simulink model "umich_2d_walking"  (R2012b)
settings: Solver=ode3  StartTime=0.0  StopTime=inf  FixedStep=sample_time  RelTol=1e-3
values from neighbouring files (symbols this model uses):
  fcut_unwrap = 50    [init_umich_2d_walking.m]
  fcut_velocity = 100    [init_umich_2d_walking.m]
  sample_time = 1/update_freq    (= 0.001)    [init_umich_2d_walking.m]
undefined symbols (not defined in the file or in its folder): BOOM_MAX_ENCODER_TICKS, boom_mount_angle, BOOM_PITCH_CAL_VALUE_RAD, BOOM_PITCH_CAL_VALUE_TICKS, BOOM_PITCH_ENCODER_RAD_PER_TICK, BOOM_ROLL_CAL_VALUE_RAD, BOOM_ROLL_CAL_VALUE_TICKS, BOOM_ROLL_ENCODER_RAD_PER_TICK, BOOM_YAW_ENCODER_RAD_PER_TICK, control_start_time, desired_torso_pitch, DiscIntNeverNeededParam, fcut_acceleration, gd, get, h_alpha, HIP_ABS_ENCODER_RAD_PER_TICK, hip_gravity_compensation, HIP_INC_ENCODER_RAD_PER_TICK, HIP_INC_MAX_ENCODER_TICKS, HIP_MOTOR_CONSTANT, HIP_MTR_GEAR_RATIO, HIP_MTR_MAX_TORQUE, i_limit_lateral, j_motor_reflected, k_leg_spring, kd_lateral, kd_pitch, kd_sea_torque, ki_lateral, kp_lateral, kp_pitch, kp_sea_torque, lateral_torque_ramp_time, LEFT_HIP_CALIB_POS, LEFT_HIP_CALIB_VAL, LEFT_MOTOR_HIP_DIRECTION, LEG1_LEG_A_CALIB_VAL, LEG1_LEG_A_RAD_PER_CNT, LEG1_LEG_B_CALIB_VAL, LEG1_LEG_B_RAD_PER_CNT, LEG1_MOTOR_A_DIRECTION, LEG1_MOTOR_B_DIRECTION, LEG1_TRAN_A_CALIB_VAL, LEG1_TRAN_A_RAD_PER_CNT, LEG1_TRAN_B_CALIB_VAL, LEG1_TRAN_B_RAD_PER_CNT, LEG2_LEG_A_CALIB_VAL, LEG2_LEG_A_RAD_PER_CNT, LEG2_LEG_B_CALIB_VAL, LEG2_LEG_B_RAD_PER_CNT, LEG2_MOTOR_A_DIRECTION, LEG2_MOTOR_B_DIRECTION, LEG2_TRAN_A_CALIB_VAL, LEG2_TRAN_A_RAD_PER_CNT, LEG2_TRAN_B_CALIB_VAL, LEG2_TRAN_B_RAD_PER_CNT, LEG_A_CALIB_LOC, LEG_B_CALIB_LOC, LEG_MOTOR_CONSTANT ... (+23)
libraries: xpcethercatlib x160, simulink x9, dspswit3 x1
(part 2 of 3)

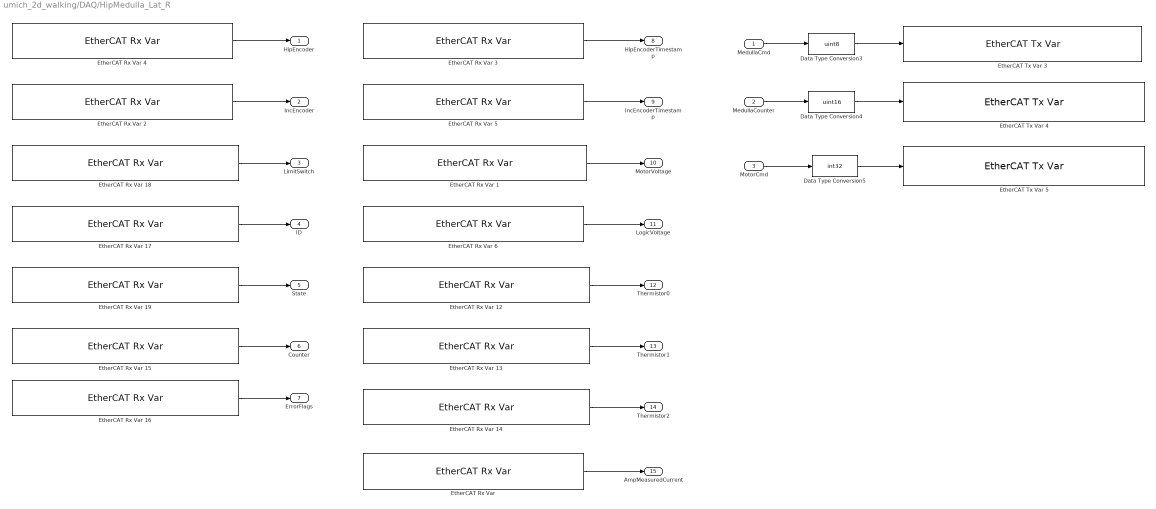
== system umich_2d_walking/DAQ/HipMedulla_Lat_R ==
  MedullaCmd : Inport
  MedullaCounter : Inport  Port=2
  MotorCmd : Inport  Port=3
  Data Type Conversion3 : DataTypeConversion  OutDataTypeStr=uint8
  Data Type Conversion4 : DataTypeConversion  OutDataTypeStr=uint16
  Data Type Conversion5 : DataTypeConversion  OutDataTypeStr=int32
  "EtherCAT Rx Var " : xpcethercatlib/EtherCAT Rx Var   Priority=2  sig_name=Box 6 (ATRIAS 2.1 Hip (Medulla 1.5)).Measured Current.Amp Measured Current  sig_offset=2352  sig_type=int16  type_size=16  sig_dim=1  device_id=0  sample_time=0.001000
  EtherCAT Rx Var 1 : xpcethercatlib/EtherCAT Rx Var   Priority=2  sig_name=Box 6 (ATRIAS 2.1 Hip (Medulla 1.5)).Power.Motor Voltage  sig_offset=2272  sig_type=uint16  type_size=16  sig_dim=1  device_id=0  sample_time=0.001000
  EtherCAT Rx Var 12 : xpcethercatlib/EtherCAT Rx Var   Priority=2  sig_name=Box 6 (ATRIAS 2.1 Hip (Medulla 1.5)).Thermistors.Thermistor 0  sig_offset=2304  sig_type=uint16  type_size=16  sig_dim=1  device_id=0  sample_time=0.001000
  EtherCAT Rx Var 13 : xpcethercatlib/EtherCAT Rx Var   Priority=2  sig_name=Box 6 (ATRIAS 2.1 Hip (Medulla 1.5)).Thermistors.Thermistor 1  sig_offset=2320  sig_type=uint16  type_size=16  sig_dim=1  device_id=0  sample_time=0.001000
  EtherCAT Rx Var 14 : xpcethercatlib/EtherCAT Rx Var   Priority=2  sig_name=Box 6 (ATRIAS 2.1 Hip (Medulla 1.5)).Thermistors.Thermistor 2  sig_offset=2336  sig_type=uint16  type_size=16  sig_dim=1  device_id=0  sample_time=0.001000
  EtherCAT Rx Var 15 : xpcethercatlib/EtherCAT Rx Var   Priority=2  sig_name=Box 6 (ATRIAS 2.1 Hip (Medulla 1.5)).uController Status.Counter  sig_offset=2200  sig_type=uint8  type_size=8  sig_dim=1  device_id=0  sample_time=0.001000
  EtherCAT Rx Var 16 : xpcethercatlib/EtherCAT Rx Var   Priority=2  sig_name=Box 6 (ATRIAS 2.1 Hip (Medulla 1.5)).uController Status.Error Flags  sig_offset=2208  sig_type=uint8  type_size=8  sig_dim=1  device_id=0  sample_time=0.001000
  EtherCAT Rx Var 17 : xpcethercatlib/EtherCAT Rx Var   Priority=2  sig_name=Box 6 (ATRIAS 2.1 Hip (Medulla 1.5)).uController Status.ID  sig_offset=2184  sig_type=uint8  type_size=8  sig_dim=1  device_id=0  sample_time=0.001000
  EtherCAT Rx Var 18 : xpcethercatlib/EtherCAT Rx Var   Priority=2  sig_name=Box 6 (ATRIAS 2.1 Hip (Medulla 1.5)).uController Status.Limit Switch  sig_offset=2216  sig_type=uint8  type_size=8  sig_dim=1  device_id=0  sample_time=0.001000
  EtherCAT Rx Var 19 : xpcethercatlib/EtherCAT Rx Var   Priority=2  sig_name=Box 6 (ATRIAS 2.1 Hip (Medulla 1.5)).uController Status.State  sig_offset=2192  sig_type=uint8  type_size=8  sig_dim=1  device_id=0  sample_time=0.001000
  EtherCAT Rx Var 2 : xpcethercatlib/EtherCAT Rx Var   Priority=2  sig_name=Box 6 (ATRIAS 2.1 Hip (Medulla 1.5)).Incremental Encoder.Incremental Encoder  sig_offset=2368  sig_type=uint16  type_size=16  sig_dim=1  device_id=0  sample_time=0.001000
  EtherCAT Rx Var 3 : xpcethercatlib/EtherCAT Rx Var   Priority=2  sig_name=Box 6 (ATRIAS 2.1 Hip (Medulla 1.5)).Hip Encoder.Timestamp  sig_offset=2256  sig_type=uint16  type_size=16  sig_dim=1  device_id=0  sample_time=0.001000
  EtherCAT Rx Var 4 : xpcethercatlib/EtherCAT Rx Var   Priority=2  sig_name=Box 6 (ATRIAS 2.1 Hip (Medulla 1.5)).Hip Encoder.Encoder  sig_offset=2224  sig_type=uint32  type_size=32  sig_dim=1  device_id=0  sample_time=0.001000
  EtherCAT Rx Var 5 : xpcethercatlib/EtherCAT Rx Var   Priority=2  sig_name=Box 6 (ATRIAS 2.1 Hip (Medulla 1.5)).Incremental Encoder.Incremental Encoder Timestamp  sig_offset=2384  sig_type=uint16  type_size=16  sig_dim=1  device_id=0  sample_time=0.001000
  EtherCAT Rx Var 6 : xpcethercatlib/EtherCAT Rx Var   Priority=2  sig_name=Box 6 (ATRIAS 2.1 Hip (Medulla 1.5)).Power.Logic Voltage  sig_offset=2288  sig_type=uint16  type_size=16  sig_dim=1  device_id=0  sample_time=0.001000
  EtherCAT Tx Var 3 : xpcethercatlib/EtherCAT Tx Var   Priority=3  sig_name=Box 6 (ATRIAS 2.1 Hip (Medulla 1.5)).uControllerInput.Command  sig_offset=2184  sig_type=uint8  type_size=8  sig_dim=1  device_id=0  sample_time=0.001000
  EtherCAT Tx Var 4 : xpcethercatlib/EtherCAT Tx Var   Priority=3  sig_name=Box 6 (ATRIAS 2.1 Hip (Medulla 1.5)).uControllerInput.Counter  sig_offset=2192  sig_type=uint16  type_size=16  sig_dim=1  device_id=0  sample_time=0.001000
  EtherCAT Tx Var 5 : xpcethercatlib/EtherCAT Tx Var   Priority=3  sig_name=Box 6 (ATRIAS 2.1 Hip (Medulla 1.5)).uControllerInput.Motor Current  sig_offset=2208  sig_type=int32  type_size=32  sig_dim=1  device_id=0  sample_time=0.001000
  HipEncoder : Outport
  IncEncoder : Outport  Port=2
  LimitSwitch : Outport  Port=3
  ID : Outport  Port=4
  State : Outport  Port=5
  Counter : Outport  Port=6
  ErrorFlags : Outport  Port=7
  HipEncoderTimestamp : Outport  Port=8
  IncEncoderTimestamp : Outport  Port=9
  MotorVoltage : Outport  Port=10
  LogicVoltage : Outport  Port=11
  Thermistor0 : Outport  Port=12
  Thermistor1 : Outport  Port=13
  Thermistor2 : Outport  Port=14
  AmpMeasuredCurrent : Outport  Port=15
  wires:
  Data Type Conversion3/1 -> EtherCAT Tx Var 3/1
  Data Type Conversion4/1 -> EtherCAT Tx Var 4/1
  Data Type Conversion5/1 -> EtherCAT Tx Var 5/1
  MedullaCmd/1 -> Data Type Conversion3/1
  MedullaCounter/1 -> Data Type Conversion4/1
  MotorCmd/1 -> Data Type Conversion5/1
  EtherCAT Rx Var 5/1 -> IncEncoderTimestamp/1
  EtherCAT Rx Var 4/1 -> HipEncoder/1
  EtherCAT Rx Var 3/1 -> HipEncoderTimestamp/1
  EtherCAT Rx Var 2/1 -> IncEncoder/1
  EtherCAT Rx Var 15/1 -> Counter/1
  EtherCAT Rx Var 17/1 -> ID/1
  EtherCAT Rx Var 18/1 -> LimitSwitch/1
  EtherCAT Rx Var 19/1 -> State/1
  EtherCAT Rx Var 16/1 -> ErrorFlags/1
  EtherCAT Rx Var 6/1 -> LogicVoltage/1
  EtherCAT Rx Var 1/1 -> MotorVoltage/1
  EtherCAT Rx Var 12/1 -> Thermistor0/1
  EtherCAT Rx Var 13/1 -> Thermistor1/1
  EtherCAT Rx Var 14/1 -> Thermistor2/1
  "EtherCAT Rx Var "/1 -> AmpMeasuredCurrent/1

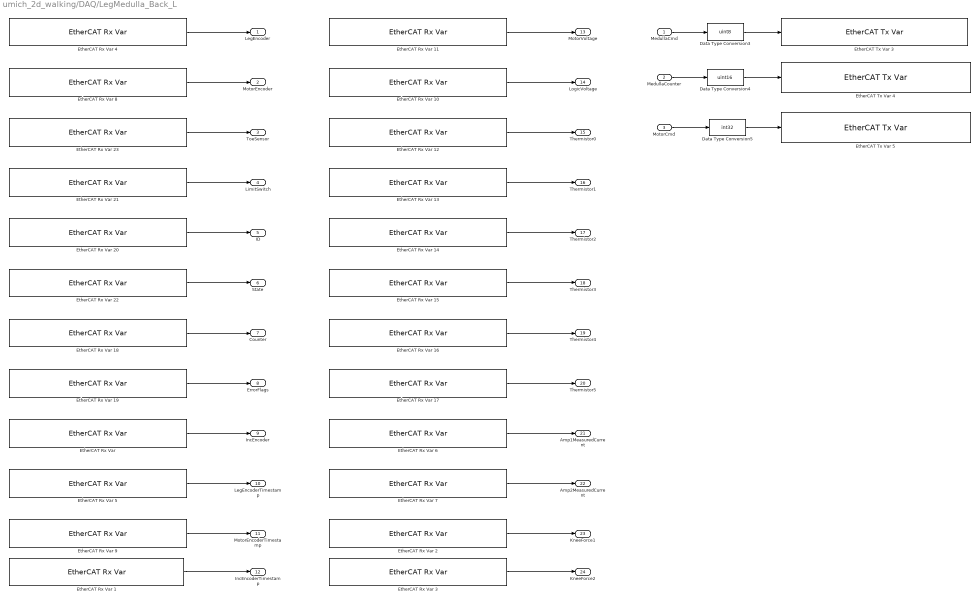
== system umich_2d_walking/DAQ/LegMedulla_Back_L ==
  MedullaCmd : Inport
  MedullaCounter : Inport  Port=2
  MotorCmd : Inport  Port=3
  Data Type Conversion3 : DataTypeConversion  OutDataTypeStr=uint8
  Data Type Conversion4 : DataTypeConversion  OutDataTypeStr=uint16
  Data Type Conversion5 : DataTypeConversion  OutDataTypeStr=int32
  "EtherCAT Rx Var " : xpcethercatlib/EtherCAT Rx Var   Priority=2  sig_name=Box 3 (ATRIAS 2.1 Leg (Medulla 1.5)).Incremental Encoder.Incremental Encoder  sig_offset=1368  sig_type=uint16  type_size=16  sig_dim=1  device_id=0  sample_time=0.001000
  EtherCAT Rx Var 1 : xpcethercatlib/EtherCAT Rx Var   Priority=2  sig_name=Box 3 (ATRIAS 2.1 Leg (Medulla 1.5)).Incremental Encoder.Incremental Encoder Timestamp  sig_offset=1384  sig_type=uint16  type_size=16  sig_dim=1  device_id=0  sample_time=0.001000
  EtherCAT Rx Var 10 : xpcethercatlib/EtherCAT Rx Var   Priority=2  sig_name=Box 3 (ATRIAS 2.1 Leg (Medulla 1.5)).Power.Logic Voltage  sig_offset=1416  sig_type=uint16  type_size=16  sig_dim=1  device_id=0  sample_time=0.001000
  EtherCAT Rx Var 11 : xpcethercatlib/EtherCAT Rx Var   Priority=2  sig_name=Box 3 (ATRIAS 2.1 Leg (Medulla 1.5)).Power.Motor Voltage  sig_offset=1400  sig_type=uint16  type_size=16  sig_dim=1  device_id=0  sample_time=0.001000
  EtherCAT Rx Var 12 : xpcethercatlib/EtherCAT Rx Var   Priority=2  sig_name=Box 3 (ATRIAS 2.1 Leg (Medulla 1.5)).Thermistors.Thermistor 0  sig_offset=1432  sig_type=uint16  type_size=16  sig_dim=1  device_id=0  sample_time=0.001000
  EtherCAT Rx Var 13 : xpcethercatlib/EtherCAT Rx Var   Priority=2  sig_name=Box 3 (ATRIAS 2.1 Leg (Medulla 1.5)).Thermistors.Thermistor 1  sig_offset=1448  sig_type=uint16  type_size=16  sig_dim=1  device_id=0  sample_time=0.001000
  EtherCAT Rx Var 14 : xpcethercatlib/EtherCAT Rx Var   Priority=2  sig_name=Box 3 (ATRIAS 2.1 Leg (Medulla 1.5)).Thermistors.Thermistor 2  sig_offset=1464  sig_type=uint16  type_size=16  sig_dim=1  device_id=0  sample_time=0.001000
  EtherCAT Rx Var 15 : xpcethercatlib/EtherCAT Rx Var   Priority=2  sig_name=Box 3 (ATRIAS 2.1 Leg (Medulla 1.5)).Thermistors.Thermistor 3  sig_offset=1480  sig_type=uint16  type_size=16  sig_dim=1  device_id=0  sample_time=0.001000
  EtherCAT Rx Var 16 : xpcethercatlib/EtherCAT Rx Var   Priority=2  sig_name=Box 3 (ATRIAS 2.1 Leg (Medulla 1.5)).Thermistors.Thermistor 4  sig_offset=1496  sig_type=uint16  type_size=16  sig_dim=1  device_id=0  sample_time=0.001000
  EtherCAT Rx Var 17 : xpcethercatlib/EtherCAT Rx Var   Priority=2  sig_name=Box 3 (ATRIAS 2.1 Leg (Medulla 1.5)).Thermistors.Thermistor 5  sig_offset=1512  sig_type=uint16  type_size=16  sig_dim=1  device_id=0  sample_time=0.001000
  EtherCAT Rx Var 18 : xpcethercatlib/EtherCAT Rx Var   Priority=2  sig_name=Box 3 (ATRIAS 2.1 Leg (Medulla 1.5)).uController Status.Counter  sig_offset=1232  sig_type=uint8  type_size=8  sig_dim=1  device_id=0  sample_time=0.001000
  EtherCAT Rx Var 19 : xpcethercatlib/EtherCAT Rx Var   Priority=2  sig_name=Box 3 (ATRIAS 2.1 Leg (Medulla 1.5)).uController Status.Error Flags  sig_offset=1240  sig_type=uint8  type_size=8  sig_dim=1  device_id=0  sample_time=0.001000
  EtherCAT Rx Var 2 : xpcethercatlib/EtherCAT Rx Var   Priority=2  sig_name=Box 3 (ATRIAS 2.1 Leg (Medulla 1.5)).Knee Force.Knee Force 1  sig_offset=1560  sig_type=uint16  type_size=16  sig_dim=1  device_id=0  sample_time=0.001000
  EtherCAT Rx Var 20 : xpcethercatlib/EtherCAT Rx Var   Priority=2  sig_name=Box 3 (ATRIAS 2.1 Leg (Medulla 1.5)).uController Status.ID  sig_offset=1216  sig_type=uint8  type_size=8  sig_dim=1  device_id=0  sample_time=0.001000
  EtherCAT Rx Var 21 : xpcethercatlib/EtherCAT Rx Var   Priority=2  sig_name=Box 3 (ATRIAS 2.1 Leg (Medulla 1.5)).uController Status.Limit Switch  sig_offset=1248  sig_type=uint8  type_size=8  sig_dim=1  device_id=0  sample_time=0.001000
  EtherCAT Rx Var 22 : xpcethercatlib/EtherCAT Rx Var   Priority=2  sig_name=Box 3 (ATRIAS 2.1 Leg (Medulla 1.5)).uController Status.State  sig_offset=1224  sig_type=uint8  type_size=8  sig_dim=1  device_id=0  sample_time=0.001000
  EtherCAT Rx Var 23 : xpcethercatlib/EtherCAT Rx Var   Priority=2  sig_name=Box 3 (ATRIAS 2.1 Leg (Medulla 1.5)).uController Status.Toe Sensor  sig_offset=1256  sig_type=uint16  type_size=16  sig_dim=1  device_id=0  sample_time=0.001000
  EtherCAT Rx Var 3 : xpcethercatlib/EtherCAT Rx Var   Priority=2  sig_name=Box 3 (ATRIAS 2.1 Leg (Medulla 1.5)).Knee Force.Knee Force 2  sig_offset=1576  sig_type=uint16  type_size=16  sig_dim=1  device_id=0  sample_time=0.001000
  EtherCAT Rx Var 4 : xpcethercatlib/EtherCAT Rx Var   Priority=2  sig_name=Box 3 (ATRIAS 2.1 Leg (Medulla 1.5)).Leg Encoder.Leg Encoder  sig_offset=1320  sig_type=uint32  type_size=32  sig_dim=1  device_id=0  sample_time=0.001000
  EtherCAT Rx Var 5 : xpcethercatlib/EtherCAT Rx Var   Priority=2  sig_name=Box 3 (ATRIAS 2.1 Leg (Medulla 1.5)).Leg Encoder.Leg Encoder Timestamp  sig_offset=1352  sig_type=uint16  type_size=16  sig_dim=1  device_id=0  sample_time=0.001000
  EtherCAT Rx Var 6 : xpcethercatlib/EtherCAT Rx Var   Priority=2  sig_name=Box 3 (ATRIAS 2.1 Leg (Medulla 1.5)).Measured Current.Amp 1 Measured Current  sig_offset=1528  sig_type=int16  type_size=16  sig_dim=1  device_id=0  sample_time=0.001000
  EtherCAT Rx Var 7 : xpcethercatlib/EtherCAT Rx Var   Priority=2  sig_name=Box 3 (ATRIAS 2.1 Leg (Medulla 1.5)).Measured Current.Amp 2 Measured Current  sig_offset=1544  sig_type=int16  type_size=16  sig_dim=1  device_id=0  sample_time=0.001000
  EtherCAT Rx Var 8 : xpcethercatlib/EtherCAT Rx Var   Priority=2  sig_name=Box 3 (ATRIAS 2.1 Leg (Medulla 1.5)).Motor Encoder.Motor Encoder  sig_offset=1272  sig_type=uint32  type_size=32  sig_dim=1  device_id=0  sample_time=0.001000
  EtherCAT Rx Var 9 : xpcethercatlib/EtherCAT Rx Var   Priority=2  sig_name=Box 3 (ATRIAS 2.1 Leg (Medulla 1.5)).Motor Encoder.Motor Encoder Timestamp  sig_offset=1304  sig_type=uint16  type_size=16  sig_dim=1  device_id=0  sample_time=0.001000
  EtherCAT Tx Var 3 : xpcethercatlib/EtherCAT Tx Var   Priority=3  sig_name=Box 3 (ATRIAS 2.1 Leg (Medulla 1.5)).uControllerInput.Command  sig_offset=1216  sig_type=uint8  type_size=8  sig_dim=1  device_id=0  sample_time=0.001000
  EtherCAT Tx Var 4 : xpcethercatlib/EtherCAT Tx Var   Priority=3  sig_name=Box 3 (ATRIAS 2.1 Leg (Medulla 1.5)).uControllerInput.Counter  sig_offset=1224  sig_type=uint16  type_size=16  sig_dim=1  device_id=0  sample_time=0.001000
  EtherCAT Tx Var 5 : xpcethercatlib/EtherCAT Tx Var   Priority=3  sig_name=Box 3 (ATRIAS 2.1 Leg (Medulla 1.5)).uControllerInput.Motor Current  sig_offset=1240  sig_type=int32  type_size=32  sig_dim=1  device_id=0  sample_time=0.001000
  LegEncoder : Outport
  MotorEncoder : Outport  Port=2
  ToeSensor : Outport  Port=3
  LimitSwitch : Outport  Port=4
  ID : Outport  Port=5
  State : Outport  Port=6
  Counter : Outport  Port=7
  ErrorFlags : Outport  Port=8
  IncEncoder : Outport  Port=9
  LegEncoderTimestamp : Outport  Port=10
  MotorEncoderTimestamp : Outport  Port=11
  IncEncoderTimestamp : Outport  Port=12
  MotorVoltage : Outport  Port=13
  LogicVoltage : Outport  Port=14
  Thermistor0 : Outport  Port=15
  Thermistor1 : Outport  Port=16
  Thermistor2 : Outport  Port=17
  Thermistor3 : Outport  Port=18
  Thermistor4 : Outport  Port=19
  Thermistor5 : Outport  Port=20
  Amp1MeasuredCurrent : Outport  Port=21
  Amp2MeasuredCurrent : Outport  Port=22
  KneeForce1 : Outport  Port=23
  KneeForce2 : Outport  Port=24
  wires:
  Data Type Conversion3/1 -> EtherCAT Tx Var 3/1
  Data Type Conversion4/1 -> EtherCAT Tx Var 4/1
  Data Type Conversion5/1 -> EtherCAT Tx Var 5/1
  "EtherCAT Rx Var "/1 -> IncEncoder/1
  EtherCAT Rx Var 1/1 -> IncEncoderTimestamp/1
  EtherCAT Rx Var 2/1 -> KneeForce1/1
  EtherCAT Rx Var 3/1 -> KneeForce2/1
  EtherCAT Rx Var 4/1 -> LegEncoder/1
  EtherCAT Rx Var 5/1 -> LegEncoderTimestamp/1
  EtherCAT Rx Var 6/1 -> Amp1MeasuredCurrent/1
  EtherCAT Rx Var 7/1 -> Amp2MeasuredCurrent/1
  EtherCAT Rx Var 8/1 -> MotorEncoder/1
  EtherCAT Rx Var 9/1 -> MotorEncoderTimestamp/1
  EtherCAT Rx Var 10/1 -> LogicVoltage/1
  EtherCAT Rx Var 11/1 -> MotorVoltage/1
  EtherCAT Rx Var 12/1 -> Thermistor0/1
  EtherCAT Rx Var 13/1 -> Thermistor1/1
  EtherCAT Rx Var 14/1 -> Thermistor2/1
  EtherCAT Rx Var 15/1 -> Thermistor3/1
  EtherCAT Rx Var 16/1 -> Thermistor4/1
  EtherCAT Rx Var 17/1 -> Thermistor5/1
  EtherCAT Rx Var 18/1 -> Counter/1
  EtherCAT Rx Var 19/1 -> ErrorFlags/1
  EtherCAT Rx Var 20/1 -> ID/1
  EtherCAT Rx Var 21/1 -> LimitSwitch/1
  EtherCAT Rx Var 22/1 -> State/1
  EtherCAT Rx Var 23/1 -> ToeSensor/1
  MedullaCmd/1 -> Data Type Conversion3/1
  MedullaCounter/1 -> Data Type Conversion4/1
  MotorCmd/1 -> Data Type Conversion5/1

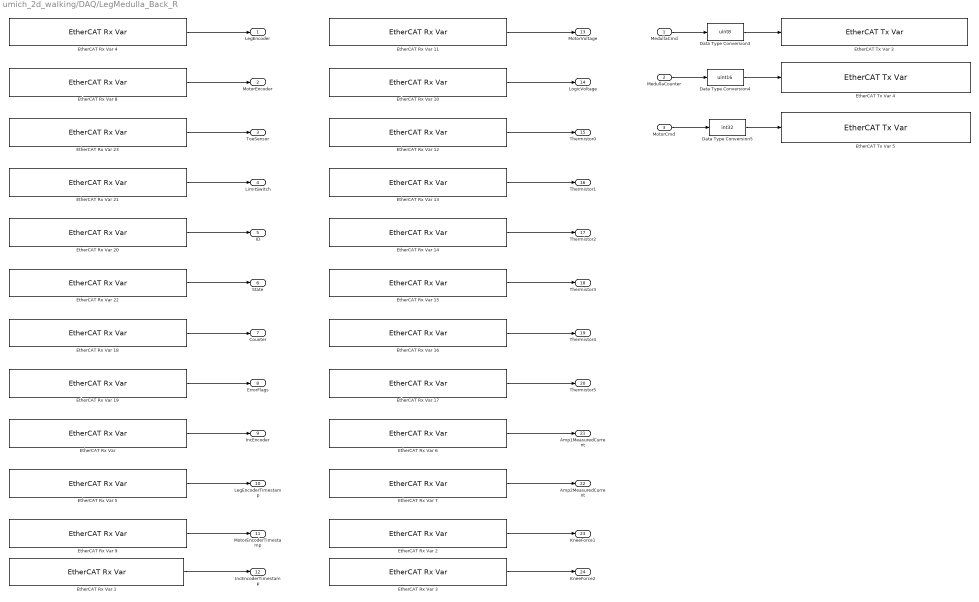
== system umich_2d_walking/DAQ/LegMedulla_Back_R ==
  MedullaCmd : Inport
  MedullaCounter : Inport  Port=2
  MotorCmd : Inport  Port=3
  Data Type Conversion3 : DataTypeConversion  OutDataTypeStr=uint8
  Data Type Conversion4 : DataTypeConversion  OutDataTypeStr=uint16
  Data Type Conversion5 : DataTypeConversion  OutDataTypeStr=int32
  "EtherCAT Rx Var " : xpcethercatlib/EtherCAT Rx Var   Priority=2  sig_name=Box 1 (ATRIAS 2.1 Leg (Medulla 1.5)).Incremental Encoder.Incremental Encoder  sig_offset=616  sig_type=uint16  type_size=16  sig_dim=1  device_id=0  sample_time=0.001000
  EtherCAT Rx Var 1 : xpcethercatlib/EtherCAT Rx Var   Priority=2  sig_name=Box 1 (ATRIAS 2.1 Leg (Medulla 1.5)).Incremental Encoder.Incremental Encoder Timestamp  sig_offset=632  sig_type=uint16  type_size=16  sig_dim=1  device_id=0  sample_time=0.001000
  EtherCAT Rx Var 10 : xpcethercatlib/EtherCAT Rx Var   Priority=2  sig_name=Box 1 (ATRIAS 2.1 Leg (Medulla 1.5)).Power.Logic Voltage  sig_offset=664  sig_type=uint16  type_size=16  sig_dim=1  device_id=0  sample_time=0.001000
  EtherCAT Rx Var 11 : xpcethercatlib/EtherCAT Rx Var   Priority=2  sig_name=Box 1 (ATRIAS 2.1 Leg (Medulla 1.5)).Power.Motor Voltage  sig_offset=648  sig_type=uint16  type_size=16  sig_dim=1  device_id=0  sample_time=0.001000
  EtherCAT Rx Var 12 : xpcethercatlib/EtherCAT Rx Var   Priority=2  sig_name=Box 1 (ATRIAS 2.1 Leg (Medulla 1.5)).Thermistors.Thermistor 0  sig_offset=680  sig_type=uint16  type_size=16  sig_dim=1  device_id=0  sample_time=0.001000
  EtherCAT Rx Var 13 : xpcethercatlib/EtherCAT Rx Var   Priority=2  sig_name=Box 1 (ATRIAS 2.1 Leg (Medulla 1.5)).Thermistors.Thermistor 1  sig_offset=696  sig_type=uint16  type_size=16  sig_dim=1  device_id=0  sample_time=0.001000
  EtherCAT Rx Var 14 : xpcethercatlib/EtherCAT Rx Var   Priority=2  sig_name=Box 1 (ATRIAS 2.1 Leg (Medulla 1.5)).Thermistors.Thermistor 2  sig_offset=712  sig_type=uint16  type_size=16  sig_dim=1  device_id=0  sample_time=0.001000
  EtherCAT Rx Var 15 : xpcethercatlib/EtherCAT Rx Var   Priority=2  sig_name=Box 1 (ATRIAS 2.1 Leg (Medulla 1.5)).Thermistors.Thermistor 3  sig_offset=728  sig_type=uint16  type_size=16  sig_dim=1  device_id=0  sample_time=0.001000
  EtherCAT Rx Var 16 : xpcethercatlib/EtherCAT Rx Var   Priority=2  sig_name=Box 1 (ATRIAS 2.1 Leg (Medulla 1.5)).Thermistors.Thermistor 4  sig_offset=744  sig_type=uint16  type_size=16  sig_dim=1  device_id=0  sample_time=0.001000
  EtherCAT Rx Var 17 : xpcethercatlib/EtherCAT Rx Var   Priority=2  sig_name=Box 1 (ATRIAS 2.1 Leg (Medulla 1.5)).Thermistors.Thermistor 5  sig_offset=760  sig_type=uint16  type_size=16  sig_dim=1  device_id=0  sample_time=0.001000
  EtherCAT Rx Var 18 : xpcethercatlib/EtherCAT Rx Var   Priority=2  sig_name=Box 1 (ATRIAS 2.1 Leg (Medulla 1.5)).uController Status.Counter  sig_offset=480  sig_type=uint8  type_size=8  sig_dim=1  device_id=0  sample_time=0.001000
  EtherCAT Rx Var 19 : xpcethercatlib/EtherCAT Rx Var   Priority=2  sig_name=Box 1 (ATRIAS 2.1 Leg (Medulla 1.5)).uController Status.Error Flags  sig_offset=488  sig_type=uint8  type_size=8  sig_dim=1  device_id=0  sample_time=0.001000
  EtherCAT Rx Var 2 : xpcethercatlib/EtherCAT Rx Var   Priority=2  sig_name=Box 1 (ATRIAS 2.1 Leg (Medulla 1.5)).Knee Force.Knee Force 1  sig_offset=808  sig_type=uint16  type_size=16  sig_dim=1  device_id=0  sample_time=0.001000
  EtherCAT Rx Var 20 : xpcethercatlib/EtherCAT Rx Var   Priority=2  sig_name=Box 1 (ATRIAS 2.1 Leg (Medulla 1.5)).uController Status.ID  sig_offset=464  sig_type=uint8  type_size=8  sig_dim=1  device_id=0  sample_time=0.001000
  EtherCAT Rx Var 21 : xpcethercatlib/EtherCAT Rx Var   Priority=2  sig_name=Box 1 (ATRIAS 2.1 Leg (Medulla 1.5)).uController Status.Limit Switch  sig_offset=496  sig_type=uint8  type_size=8  sig_dim=1  device_id=0  sample_time=0.001000
  EtherCAT Rx Var 22 : xpcethercatlib/EtherCAT Rx Var   Priority=2  sig_name=Box 1 (ATRIAS 2.1 Leg (Medulla 1.5)).uController Status.State  sig_offset=472  sig_type=uint8  type_size=8  sig_dim=1  device_id=0  sample_time=0.001000
  EtherCAT Rx Var 23 : xpcethercatlib/EtherCAT Rx Var   Priority=2  sig_name=Box 1 (ATRIAS 2.1 Leg (Medulla 1.5)).uController Status.Toe Sensor  sig_offset=504  sig_type=uint16  type_size=16  sig_dim=1  device_id=0  sample_time=0.001000
  EtherCAT Rx Var 3 : xpcethercatlib/EtherCAT Rx Var   Priority=2  sig_name=Box 1 (ATRIAS 2.1 Leg (Medulla 1.5)).Knee Force.Knee Force 2  sig_offset=824  sig_type=uint16  type_size=16  sig_dim=1  device_id=0  sample_time=0.001000
  EtherCAT Rx Var 4 : xpcethercatlib/EtherCAT Rx Var   Priority=2  sig_name=Box 1 (ATRIAS 2.1 Leg (Medulla 1.5)).Leg Encoder.Leg Encoder  sig_offset=568  sig_type=uint32  type_size=32  sig_dim=1  device_id=0  sample_time=0.001000
  EtherCAT Rx Var 5 : xpcethercatlib/EtherCAT Rx Var   Priority=2  sig_name=Box 1 (ATRIAS 2.1 Leg (Medulla 1.5)).Leg Encoder.Leg Encoder Timestamp  sig_offset=600  sig_type=uint16  type_size=16  sig_dim=1  device_id=0  sample_time=0.001000
  EtherCAT Rx Var 6 : xpcethercatlib/EtherCAT Rx Var   Priority=2  sig_name=Box 1 (ATRIAS 2.1 Leg (Medulla 1.5)).Measured Current.Amp 1 Measured Current  sig_offset=776  sig_type=int16  type_size=16  sig_dim=1  device_id=0  sample_time=0.001000
  EtherCAT Rx Var 7 : xpcethercatlib/EtherCAT Rx Var   Priority=2  sig_name=Box 1 (ATRIAS 2.1 Leg (Medulla 1.5)).Measured Current.Amp 2 Measured Current  sig_offset=792  sig_type=int16  type_size=16  sig_dim=1  device_id=0  sample_time=0.001000
  EtherCAT Rx Var 8 : xpcethercatlib/EtherCAT Rx Var   Priority=2  sig_name=Box 1 (ATRIAS 2.1 Leg (Medulla 1.5)).Motor Encoder.Motor Encoder  sig_offset=520  sig_type=uint32  type_size=32  sig_dim=1  device_id=0  sample_time=0.001000
  EtherCAT Rx Var 9 : xpcethercatlib/EtherCAT Rx Var   Priority=2  sig_name=Box 1 (ATRIAS 2.1 Leg (Medulla 1.5)).Motor Encoder.Motor Encoder Timestamp  sig_offset=552  sig_type=uint16  type_size=16  sig_dim=1  device_id=0  sample_time=0.001000
  EtherCAT Tx Var 3 : xpcethercatlib/EtherCAT Tx Var   Priority=3  sig_name=Box 1 (ATRIAS 2.1 Leg (Medulla 1.5)).uControllerInput.Command  sig_offset=464  sig_type=uint8  type_size=8  sig_dim=1  device_id=0  sample_time=0.001000
  EtherCAT Tx Var 4 : xpcethercatlib/EtherCAT Tx Var   Priority=3  sig_name=Box 1 (ATRIAS 2.1 Leg (Medulla 1.5)).uControllerInput.Counter  sig_offset=472  sig_type=uint16  type_size=16  sig_dim=1  device_id=0  sample_time=0.001000
  EtherCAT Tx Var 5 : xpcethercatlib/EtherCAT Tx Var   Priority=3  sig_name=Box 1 (ATRIAS 2.1 Leg (Medulla 1.5)).uControllerInput.Motor Current  sig_offset=488  sig_type=int32  type_size=32  sig_dim=1  device_id=0  sample_time=0.001000
  LegEncoder : Outport
  MotorEncoder : Outport  Port=2
  ToeSensor : Outport  Port=3
  LimitSwitch : Outport  Port=4
  ID : Outport  Port=5
  State : Outport  Port=6
  Counter : Outport  Port=7
  ErrorFlags : Outport  Port=8
  IncEncoder : Outport  Port=9
  LegEncoderTimestamp : Outport  Port=10
  MotorEncoderTimestamp : Outport  Port=11
  IncEncoderTimestamp : Outport  Port=12
  MotorVoltage : Outport  Port=13
  LogicVoltage : Outport  Port=14
  Thermistor0 : Outport  Port=15
  Thermistor1 : Outport  Port=16
  Thermistor2 : Outport  Port=17
  Thermistor3 : Outport  Port=18
  Thermistor4 : Outport  Port=19
  Thermistor5 : Outport  Port=20
  Amp1MeasuredCurrent : Outport  Port=21
  Amp2MeasuredCurrent : Outport  Port=22
  KneeForce1 : Outport  Port=23
  KneeForce2 : Outport  Port=24
  wires:
  Data Type Conversion3/1 -> EtherCAT Tx Var 3/1
  Data Type Conversion4/1 -> EtherCAT Tx Var 4/1
  Data Type Conversion5/1 -> EtherCAT Tx Var 5/1
  "EtherCAT Rx Var "/1 -> IncEncoder/1
  EtherCAT Rx Var 1/1 -> IncEncoderTimestamp/1
  EtherCAT Rx Var 2/1 -> KneeForce1/1
  EtherCAT Rx Var 3/1 -> KneeForce2/1
  EtherCAT Rx Var 4/1 -> LegEncoder/1
  EtherCAT Rx Var 5/1 -> LegEncoderTimestamp/1
  EtherCAT Rx Var 6/1 -> Amp1MeasuredCurrent/1
  EtherCAT Rx Var 7/1 -> Amp2MeasuredCurrent/1
  EtherCAT Rx Var 8/1 -> MotorEncoder/1
  EtherCAT Rx Var 9/1 -> MotorEncoderTimestamp/1
  EtherCAT Rx Var 10/1 -> LogicVoltage/1
  EtherCAT Rx Var 11/1 -> MotorVoltage/1
  EtherCAT Rx Var 12/1 -> Thermistor0/1
  EtherCAT Rx Var 13/1 -> Thermistor1/1
  EtherCAT Rx Var 14/1 -> Thermistor2/1
  EtherCAT Rx Var 15/1 -> Thermistor3/1
  EtherCAT Rx Var 16/1 -> Thermistor4/1
  EtherCAT Rx Var 17/1 -> Thermistor5/1
  EtherCAT Rx Var 18/1 -> Counter/1
  EtherCAT Rx Var 19/1 -> ErrorFlags/1
  EtherCAT Rx Var 20/1 -> ID/1
  EtherCAT Rx Var 21/1 -> LimitSwitch/1
  EtherCAT Rx Var 22/1 -> State/1
  EtherCAT Rx Var 23/1 -> ToeSensor/1
  MedullaCmd/1 -> Data Type Conversion3/1
  MedullaCounter/1 -> Data Type Conversion4/1
  MotorCmd/1 -> Data Type Conversion5/1

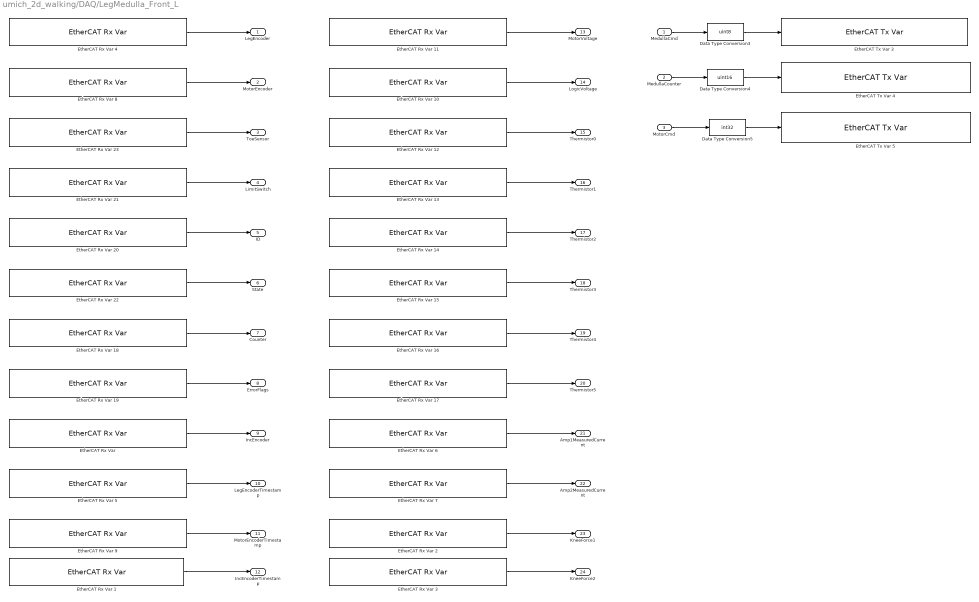
== system umich_2d_walking/DAQ/LegMedulla_Front_L ==
  MedullaCmd : Inport
  MedullaCounter : Inport  Port=2
  MotorCmd : Inport  Port=3
  Data Type Conversion3 : DataTypeConversion  OutDataTypeStr=uint8
  Data Type Conversion4 : DataTypeConversion  OutDataTypeStr=uint16
  Data Type Conversion5 : DataTypeConversion  OutDataTypeStr=int32
  "EtherCAT Rx Var " : xpcethercatlib/EtherCAT Rx Var   Priority=2  sig_name=Box 4 (ATRIAS 2.1 Leg (Medulla 1.5)).Incremental Encoder.Incremental Encoder  sig_offset=1744  sig_type=uint16  type_size=16  sig_dim=1  device_id=0  sample_time=0.001000
  EtherCAT Rx Var 1 : xpcethercatlib/EtherCAT Rx Var   Priority=2  sig_name=Box 4 (ATRIAS 2.1 Leg (Medulla 1.5)).Incremental Encoder.Incremental Encoder Timestamp  sig_offset=1760  sig_type=uint16  type_size=16  sig_dim=1  device_id=0  sample_time=0.001000
  EtherCAT Rx Var 10 : xpcethercatlib/EtherCAT Rx Var   Priority=2  sig_name=Box 4 (ATRIAS 2.1 Leg (Medulla 1.5)).Power.Logic Voltage  sig_offset=1792  sig_type=uint16  type_size=16  sig_dim=1  device_id=0  sample_time=0.001000
  EtherCAT Rx Var 11 : xpcethercatlib/EtherCAT Rx Var   Priority=2  sig_name=Box 4 (ATRIAS 2.1 Leg (Medulla 1.5)).Power.Motor Voltage  sig_offset=1776  sig_type=uint16  type_size=16  sig_dim=1  device_id=0  sample_time=0.001000
  EtherCAT Rx Var 12 : xpcethercatlib/EtherCAT Rx Var   Priority=2  sig_name=Box 4 (ATRIAS 2.1 Leg (Medulla 1.5)).Thermistors.Thermistor 0  sig_offset=1808  sig_type=uint16  type_size=16  sig_dim=1  device_id=0  sample_time=0.001000
  EtherCAT Rx Var 13 : xpcethercatlib/EtherCAT Rx Var   Priority=2  sig_name=Box 4 (ATRIAS 2.1 Leg (Medulla 1.5)).Thermistors.Thermistor 1  sig_offset=1824  sig_type=uint16  type_size=16  sig_dim=1  device_id=0  sample_time=0.001000
  EtherCAT Rx Var 14 : xpcethercatlib/EtherCAT Rx Var   Priority=2  sig_name=Box 4 (ATRIAS 2.1 Leg (Medulla 1.5)).Thermistors.Thermistor 2  sig_offset=1840  sig_type=uint16  type_size=16  sig_dim=1  device_id=0  sample_time=0.001000
  EtherCAT Rx Var 15 : xpcethercatlib/EtherCAT Rx Var   Priority=2  sig_name=Box 4 (ATRIAS 2.1 Leg (Medulla 1.5)).Thermistors.Thermistor 3  sig_offset=1856  sig_type=uint16  type_size=16  sig_dim=1  device_id=0  sample_time=0.001000
  EtherCAT Rx Var 16 : xpcethercatlib/EtherCAT Rx Var   Priority=2  sig_name=Box 4 (ATRIAS 2.1 Leg (Medulla 1.5)).Thermistors.Thermistor 4  sig_offset=1872  sig_type=uint16  type_size=16  sig_dim=1  device_id=0  sample_time=0.001000
  EtherCAT Rx Var 17 : xpcethercatlib/EtherCAT Rx Var   Priority=2  sig_name=Box 4 (ATRIAS 2.1 Leg (Medulla 1.5)).Thermistors.Thermistor 5  sig_offset=1888  sig_type=uint16  type_size=16  sig_dim=1  device_id=0  sample_time=0.001000
  EtherCAT Rx Var 18 : xpcethercatlib/EtherCAT Rx Var   Priority=2  sig_name=Box 4 (ATRIAS 2.1 Leg (Medulla 1.5)).uController Status.Counter  sig_offset=1608  sig_type=uint8  type_size=8  sig_dim=1  device_id=0  sample_time=0.001000
  EtherCAT Rx Var 19 : xpcethercatlib/EtherCAT Rx Var   Priority=2  sig_name=Box 4 (ATRIAS 2.1 Leg (Medulla 1.5)).uController Status.Error Flags  sig_offset=1616  sig_type=uint8  type_size=8  sig_dim=1  device_id=0  sample_time=0.001000
  EtherCAT Rx Var 2 : xpcethercatlib/EtherCAT Rx Var   Priority=2  sig_name=Box 4 (ATRIAS 2.1 Leg (Medulla 1.5)).Knee Force.Knee Force 1  sig_offset=1936  sig_type=uint16  type_size=16  sig_dim=1  device_id=0  sample_time=0.001000
  EtherCAT Rx Var 20 : xpcethercatlib/EtherCAT Rx Var   Priority=2  sig_name=Box 4 (ATRIAS 2.1 Leg (Medulla 1.5)).uController Status.ID  sig_offset=1592  sig_type=uint8  type_size=8  sig_dim=1  device_id=0  sample_time=0.001000
  EtherCAT Rx Var 21 : xpcethercatlib/EtherCAT Rx Var   Priority=2  sig_name=Box 4 (ATRIAS 2.1 Leg (Medulla 1.5)).uController Status.Limit Switch  sig_offset=1624  sig_type=uint8  type_size=8  sig_dim=1  device_id=0  sample_time=0.001000
  EtherCAT Rx Var 22 : xpcethercatlib/EtherCAT Rx Var   Priority=2  sig_name=Box 4 (ATRIAS 2.1 Leg (Medulla 1.5)).uController Status.State  sig_offset=1600  sig_type=uint8  type_size=8  sig_dim=1  device_id=0  sample_time=0.001000
  EtherCAT Rx Var 23 : xpcethercatlib/EtherCAT Rx Var   Priority=2  sig_name=Box 4 (ATRIAS 2.1 Leg (Medulla 1.5)).uController Status.Toe Sensor  sig_offset=1632  sig_type=uint16  type_size=16  sig_dim=1  device_id=0  sample_time=0.001000
  EtherCAT Rx Var 3 : xpcethercatlib/EtherCAT Rx Var   Priority=2  sig_name=Box 4 (ATRIAS 2.1 Leg (Medulla 1.5)).Knee Force.Knee Force 2  sig_offset=1952  sig_type=uint16  type_size=16  sig_dim=1  device_id=0  sample_time=0.001000
  EtherCAT Rx Var 4 : xpcethercatlib/EtherCAT Rx Var   Priority=2  sig_name=Box 4 (ATRIAS 2.1 Leg (Medulla 1.5)).Leg Encoder.Leg Encoder  sig_offset=1696  sig_type=uint32  type_size=32  sig_dim=1  device_id=0  sample_time=0.001000
  EtherCAT Rx Var 5 : xpcethercatlib/EtherCAT Rx Var   Priority=2  sig_name=Box 4 (ATRIAS 2.1 Leg (Medulla 1.5)).Leg Encoder.Leg Encoder Timestamp  sig_offset=1728  sig_type=uint16  type_size=16  sig_dim=1  device_id=0  sample_time=0.001000
  EtherCAT Rx Var 6 : xpcethercatlib/EtherCAT Rx Var   Priority=2  sig_name=Box 4 (ATRIAS 2.1 Leg (Medulla 1.5)).Measured Current.Amp 1 Measured Current  sig_offset=1904  sig_type=int16  type_size=16  sig_dim=1  device_id=0  sample_time=0.001000
  EtherCAT Rx Var 7 : xpcethercatlib/EtherCAT Rx Var   Priority=2  sig_name=Box 4 (ATRIAS 2.1 Leg (Medulla 1.5)).Measured Current.Amp 2 Measured Current  sig_offset=1920  sig_type=int16  type_size=16  sig_dim=1  device_id=0  sample_time=0.001000
  EtherCAT Rx Var 8 : xpcethercatlib/EtherCAT Rx Var   Priority=2  sig_name=Box 4 (ATRIAS 2.1 Leg (Medulla 1.5)).Motor Encoder.Motor Encoder  sig_offset=1648  sig_type=uint32  type_size=32  sig_dim=1  device_id=0  sample_time=0.001000
  EtherCAT Rx Var 9 : xpcethercatlib/EtherCAT Rx Var   Priority=2  sig_name=Box 4 (ATRIAS 2.1 Leg (Medulla 1.5)).Motor Encoder.Motor Encoder Timestamp  sig_offset=1680  sig_type=uint16  type_size=16  sig_dim=1  device_id=0  sample_time=0.001000
  EtherCAT Tx Var 3 : xpcethercatlib/EtherCAT Tx Var   Priority=3  sig_name=Box 4 (ATRIAS 2.1 Leg (Medulla 1.5)).uControllerInput.Command  sig_offset=1592  sig_type=uint8  type_size=8  sig_dim=1  device_id=0  sample_time=0.001000
  EtherCAT Tx Var 4 : xpcethercatlib/EtherCAT Tx Var   Priority=3  sig_name=Box 4 (ATRIAS 2.1 Leg (Medulla 1.5)).uControllerInput.Counter  sig_offset=1600  sig_type=uint16  type_size=16  sig_dim=1  device_id=0  sample_time=0.001000
  EtherCAT Tx Var 5 : xpcethercatlib/EtherCAT Tx Var   Priority=3  sig_name=Box 4 (ATRIAS 2.1 Leg (Medulla 1.5)).uControllerInput.Motor Current  sig_offset=1616  sig_type=int32  type_size=32  sig_dim=1  device_id=0  sample_time=0.001000
  LegEncoder : Outport
  MotorEncoder : Outport  Port=2
  ToeSensor : Outport  Port=3
  LimitSwitch : Outport  Port=4
  ID : Outport  Port=5
  State : Outport  Port=6
  Counter : Outport  Port=7
  ErrorFlags : Outport  Port=8
  IncEncoder : Outport  Port=9
  LegEncoderTimestamp : Outport  Port=10
  MotorEncoderTimestamp : Outport  Port=11
  IncEncoderTimestamp : Outport  Port=12
  MotorVoltage : Outport  Port=13
  LogicVoltage : Outport  Port=14
  Thermistor0 : Outport  Port=15
  Thermistor1 : Outport  Port=16
  Thermistor2 : Outport  Port=17
  Thermistor3 : Outport  Port=18
  Thermistor4 : Outport  Port=19
  Thermistor5 : Outport  Port=20
  Amp1MeasuredCurrent : Outport  Port=21
  Amp2MeasuredCurrent : Outport  Port=22
  KneeForce1 : Outport  Port=23
  KneeForce2 : Outport  Port=24
  wires:
  Data Type Conversion3/1 -> EtherCAT Tx Var 3/1
  Data Type Conversion4/1 -> EtherCAT Tx Var 4/1
  Data Type Conversion5/1 -> EtherCAT Tx Var 5/1
  "EtherCAT Rx Var "/1 -> IncEncoder/1
  EtherCAT Rx Var 1/1 -> IncEncoderTimestamp/1
  EtherCAT Rx Var 2/1 -> KneeForce1/1
  EtherCAT Rx Var 3/1 -> KneeForce2/1
  EtherCAT Rx Var 4/1 -> LegEncoder/1
  EtherCAT Rx Var 5/1 -> LegEncoderTimestamp/1
  EtherCAT Rx Var 6/1 -> Amp1MeasuredCurrent/1
  EtherCAT Rx Var 7/1 -> Amp2MeasuredCurrent/1
  EtherCAT Rx Var 8/1 -> MotorEncoder/1
  EtherCAT Rx Var 9/1 -> MotorEncoderTimestamp/1
  EtherCAT Rx Var 10/1 -> LogicVoltage/1
  EtherCAT Rx Var 11/1 -> MotorVoltage/1
  EtherCAT Rx Var 12/1 -> Thermistor0/1
  EtherCAT Rx Var 13/1 -> Thermistor1/1
  EtherCAT Rx Var 14/1 -> Thermistor2/1
  EtherCAT Rx Var 15/1 -> Thermistor3/1
  EtherCAT Rx Var 16/1 -> Thermistor4/1
  EtherCAT Rx Var 17/1 -> Thermistor5/1
  EtherCAT Rx Var 18/1 -> Counter/1
  EtherCAT Rx Var 19/1 -> ErrorFlags/1
  EtherCAT Rx Var 20/1 -> ID/1
  EtherCAT Rx Var 21/1 -> LimitSwitch/1
  EtherCAT Rx Var 22/1 -> State/1
  EtherCAT Rx Var 23/1 -> ToeSensor/1
  MedullaCmd/1 -> Data Type Conversion3/1
  MedullaCounter/1 -> Data Type Conversion4/1
  MotorCmd/1 -> Data Type Conversion5/1

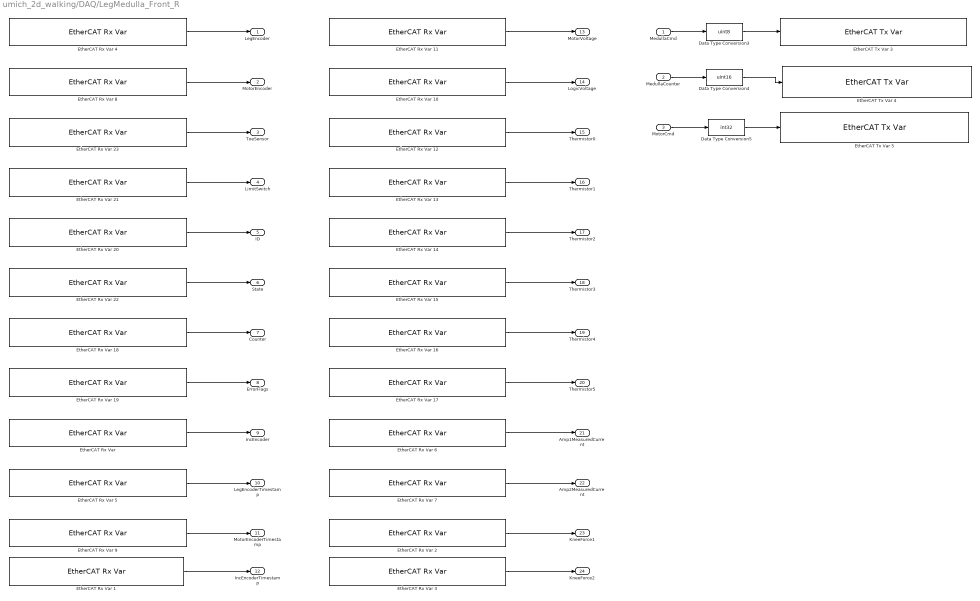
== system umich_2d_walking/DAQ/LegMedulla_Front_R ==
  MedullaCmd : Inport
  MedullaCounter : Inport  Port=2
  MotorCmd : Inport  Port=3
  Data Type Conversion3 : DataTypeConversion  OutDataTypeStr=uint8
  Data Type Conversion4 : DataTypeConversion  OutDataTypeStr=uint16
  Data Type Conversion5 : DataTypeConversion  OutDataTypeStr=int32
  "EtherCAT Rx Var " : xpcethercatlib/EtherCAT Rx Var   Priority=2  sig_name=Box 2 (ATRIAS 2.1 Leg (Medulla 1.5)).Incremental Encoder.Incremental Encoder  sig_offset=992  sig_type=uint16  type_size=16  sig_dim=1  device_id=0  sample_time=0.001000
  EtherCAT Rx Var 1 : xpcethercatlib/EtherCAT Rx Var   Priority=2  sig_name=Box 2 (ATRIAS 2.1 Leg (Medulla 1.5)).Incremental Encoder.Incremental Encoder Timestamp  sig_offset=1008  sig_type=uint16  type_size=16  sig_dim=1  device_id=0  sample_time=0.001000
  EtherCAT Rx Var 10 : xpcethercatlib/EtherCAT Rx Var   Priority=2  sig_name=Box 2 (ATRIAS 2.1 Leg (Medulla 1.5)).Power.Logic Voltage  sig_offset=1040  sig_type=uint16  type_size=16  sig_dim=1  device_id=0  sample_time=0.001000
  EtherCAT Rx Var 11 : xpcethercatlib/EtherCAT Rx Var   Priority=2  sig_name=Box 2 (ATRIAS 2.1 Leg (Medulla 1.5)).Power.Motor Voltage  sig_offset=1024  sig_type=uint16  type_size=16  sig_dim=1  device_id=0  sample_time=0.001000
  EtherCAT Rx Var 12 : xpcethercatlib/EtherCAT Rx Var   Priority=2  sig_name=Box 2 (ATRIAS 2.1 Leg (Medulla 1.5)).Thermistors.Thermistor 0  sig_offset=1056  sig_type=uint16  type_size=16  sig_dim=1  device_id=0  sample_time=0.001000
  EtherCAT Rx Var 13 : xpcethercatlib/EtherCAT Rx Var   Priority=2  sig_name=Box 2 (ATRIAS 2.1 Leg (Medulla 1.5)).Thermistors.Thermistor 1  sig_offset=1072  sig_type=uint16  type_size=16  sig_dim=1  device_id=0  sample_time=0.001000
  EtherCAT Rx Var 14 : xpcethercatlib/EtherCAT Rx Var   Priority=2  sig_name=Box 2 (ATRIAS 2.1 Leg (Medulla 1.5)).Thermistors.Thermistor 2  sig_offset=1088  sig_type=uint16  type_size=16  sig_dim=1  device_id=0  sample_time=0.001000
  EtherCAT Rx Var 15 : xpcethercatlib/EtherCAT Rx Var   Priority=2  sig_name=Box 2 (ATRIAS 2.1 Leg (Medulla 1.5)).Thermistors.Thermistor 3  sig_offset=1104  sig_type=uint16  type_size=16  sig_dim=1  device_id=0  sample_time=0.001000
  EtherCAT Rx Var 16 : xpcethercatlib/EtherCAT Rx Var   Priority=2  sig_name=Box 2 (ATRIAS 2.1 Leg (Medulla 1.5)).Thermistors.Thermistor 4  sig_offset=1120  sig_type=uint16  type_size=16  sig_dim=1  device_id=0  sample_time=0.001000
  EtherCAT Rx Var 17 : xpcethercatlib/EtherCAT Rx Var   Priority=2  sig_name=Box 2 (ATRIAS 2.1 Leg (Medulla 1.5)).Thermistors.Thermistor 5  sig_offset=1136  sig_type=uint16  type_size=16  sig_dim=1  device_id=0  sample_time=0.001000
  EtherCAT Rx Var 18 : xpcethercatlib/EtherCAT Rx Var   Priority=2  sig_name=Box 2 (ATRIAS 2.1 Leg (Medulla 1.5)).uController Status.Counter  sig_offset=856  sig_type=uint8  type_size=8  sig_dim=1  device_id=0  sample_time=0.001000
  EtherCAT Rx Var 19 : xpcethercatlib/EtherCAT Rx Var   Priority=2  sig_name=Box 2 (ATRIAS 2.1 Leg (Medulla 1.5)).uController Status.Error Flags  sig_offset=864  sig_type=uint8  type_size=8  sig_dim=1  device_id=0  sample_time=0.001000
  EtherCAT Rx Var 2 : xpcethercatlib/EtherCAT Rx Var   Priority=2  sig_name=Box 2 (ATRIAS 2.1 Leg (Medulla 1.5)).Knee Force.Knee Force 1  sig_offset=1184  sig_type=uint16  type_size=16  sig_dim=1  device_id=0  sample_time=0.001000
  EtherCAT Rx Var 20 : xpcethercatlib/EtherCAT Rx Var   Priority=2  sig_name=Box 2 (ATRIAS 2.1 Leg (Medulla 1.5)).uController Status.ID  sig_offset=840  sig_type=uint8  type_size=8  sig_dim=1  device_id=0  sample_time=0.001000
  EtherCAT Rx Var 21 : xpcethercatlib/EtherCAT Rx Var   Priority=2  sig_name=Box 2 (ATRIAS 2.1 Leg (Medulla 1.5)).uController Status.Limit Switch  sig_offset=872  sig_type=uint8  type_size=8  sig_dim=1  device_id=0  sample_time=0.001000
  EtherCAT Rx Var 22 : xpcethercatlib/EtherCAT Rx Var   Priority=2  sig_name=Box 2 (ATRIAS 2.1 Leg (Medulla 1.5)).uController Status.State  sig_offset=848  sig_type=uint8  type_size=8  sig_dim=1  device_id=0  sample_time=0.001000
  EtherCAT Rx Var 23 : xpcethercatlib/EtherCAT Rx Var   Priority=2  sig_name=Box 2 (ATRIAS 2.1 Leg (Medulla 1.5)).uController Status.Toe Sensor  sig_offset=880  sig_type=uint16  type_size=16  sig_dim=1  device_id=0  sample_time=0.001000
  EtherCAT Rx Var 3 : xpcethercatlib/EtherCAT Rx Var   Priority=2  sig_name=Box 2 (ATRIAS 2.1 Leg (Medulla 1.5)).Knee Force.Knee Force 2  sig_offset=1200  sig_type=uint16  type_size=16  sig_dim=1  device_id=0  sample_time=0.001000
  EtherCAT Rx Var 4 : xpcethercatlib/EtherCAT Rx Var   Priority=2  sig_name=Box 2 (ATRIAS 2.1 Leg (Medulla 1.5)).Leg Encoder.Leg Encoder  sig_offset=944  sig_type=uint32  type_size=32  sig_dim=1  device_id=0  sample_time=0.001000
  EtherCAT Rx Var 5 : xpcethercatlib/EtherCAT Rx Var   Priority=2  sig_name=Box 2 (ATRIAS 2.1 Leg (Medulla 1.5)).Leg Encoder.Leg Encoder Timestamp  sig_offset=976  sig_type=uint16  type_size=16  sig_dim=1  device_id=0  sample_time=0.001000
  EtherCAT Rx Var 6 : xpcethercatlib/EtherCAT Rx Var   Priority=2  sig_name=Box 2 (ATRIAS 2.1 Leg (Medulla 1.5)).Measured Current.Amp 1 Measured Current  sig_offset=1152  sig_type=int16  type_size=16  sig_dim=1  device_id=0  sample_time=0.001000
  EtherCAT Rx Var 7 : xpcethercatlib/EtherCAT Rx Var   Priority=2  sig_name=Box 2 (ATRIAS 2.1 Leg (Medulla 1.5)).Measured Current.Amp 2 Measured Current  sig_offset=1168  sig_type=int16  type_size=16  sig_dim=1  device_id=0  sample_time=0.001000
  EtherCAT Rx Var 8 : xpcethercatlib/EtherCAT Rx Var   Priority=2  sig_name=Box 2 (ATRIAS 2.1 Leg (Medulla 1.5)).Motor Encoder.Motor Encoder  sig_offset=896  sig_type=uint32  type_size=32  sig_dim=1  device_id=0  sample_time=0.001000
  EtherCAT Rx Var 9 : xpcethercatlib/EtherCAT Rx Var   Priority=2  sig_name=Box 2 (ATRIAS 2.1 Leg (Medulla 1.5)).Motor Encoder.Motor Encoder Timestamp  sig_offset=928  sig_type=uint16  type_size=16  sig_dim=1  device_id=0  sample_time=0.001000
  EtherCAT Tx Var 3 : xpcethercatlib/EtherCAT Tx Var   Priority=3  sig_name=Box 2 (ATRIAS 2.1 Leg (Medulla 1.5)).uControllerInput.Command  sig_offset=840  sig_type=uint8  type_size=8  sig_dim=1  device_id=0  sample_time=0.001000
  EtherCAT Tx Var 4 : xpcethercatlib/EtherCAT Tx Var   Priority=3  sig_name=Box 2 (ATRIAS 2.1 Leg (Medulla 1.5)).uControllerInput.Counter  sig_offset=848  sig_type=uint16  type_size=16  sig_dim=1  device_id=0  sample_time=0.001000
  EtherCAT Tx Var 5 : xpcethercatlib/EtherCAT Tx Var   Priority=3  sig_name=Box 2 (ATRIAS 2.1 Leg (Medulla 1.5)).uControllerInput.Motor Current  sig_offset=864  sig_type=int32  type_size=32  sig_dim=1  device_id=0  sample_time=0.001000
  LegEncoder : Outport
  MotorEncoder : Outport  Port=2
  ToeSensor : Outport  Port=3
  LimitSwitch : Outport  Port=4
  ID : Outport  Port=5
  State : Outport  Port=6
  Counter : Outport  Port=7
  ErrorFlags : Outport  Port=8
  IncEncoder : Outport  Port=9
  LegEncoderTimestamp : Outport  Port=10
  MotorEncoderTimestamp : Outport  Port=11
  IncEncoderTimestamp : Outport  Port=12
  MotorVoltage : Outport  Port=13
  LogicVoltage : Outport  Port=14
  Thermistor0 : Outport  Port=15
  Thermistor1 : Outport  Port=16
  Thermistor2 : Outport  Port=17
  Thermistor3 : Outport  Port=18
  Thermistor4 : Outport  Port=19
  Thermistor5 : Outport  Port=20
  Amp1MeasuredCurrent : Outport  Port=21
  Amp2MeasuredCurrent : Outport  Port=22
  KneeForce1 : Outport  Port=23
  KneeForce2 : Outport  Port=24
  wires:
  Data Type Conversion3/1 -> EtherCAT Tx Var 3/1
  Data Type Conversion4/1 -> EtherCAT Tx Var 4/1
  Data Type Conversion5/1 -> EtherCAT Tx Var 5/1
  "EtherCAT Rx Var "/1 -> IncEncoder/1
  EtherCAT Rx Var 1/1 -> IncEncoderTimestamp/1
  EtherCAT Rx Var 2/1 -> KneeForce1/1
  EtherCAT Rx Var 3/1 -> KneeForce2/1
  EtherCAT Rx Var 4/1 -> LegEncoder/1
  EtherCAT Rx Var 5/1 -> LegEncoderTimestamp/1
  EtherCAT Rx Var 6/1 -> Amp1MeasuredCurrent/1
  EtherCAT Rx Var 7/1 -> Amp2MeasuredCurrent/1
  EtherCAT Rx Var 8/1 -> MotorEncoder/1
  EtherCAT Rx Var 9/1 -> MotorEncoderTimestamp/1
  EtherCAT Rx Var 10/1 -> LogicVoltage/1
  EtherCAT Rx Var 11/1 -> MotorVoltage/1
  EtherCAT Rx Var 12/1 -> Thermistor0/1
  EtherCAT Rx Var 13/1 -> Thermistor1/1
  EtherCAT Rx Var 14/1 -> Thermistor2/1
  EtherCAT Rx Var 15/1 -> Thermistor3/1
  EtherCAT Rx Var 16/1 -> Thermistor4/1
  EtherCAT Rx Var 17/1 -> Thermistor5/1
  EtherCAT Rx Var 18/1 -> Counter/1
  EtherCAT Rx Var 19/1 -> ErrorFlags/1
  EtherCAT Rx Var 20/1 -> ID/1
  EtherCAT Rx Var 21/1 -> LimitSwitch/1
  EtherCAT Rx Var 22/1 -> State/1
  EtherCAT Rx Var 23/1 -> ToeSensor/1
  MedullaCmd/1 -> Data Type Conversion3/1
  MedullaCounter/1 -> Data Type Conversion4/1
  MotorCmd/1 -> Data Type Conversion5/1

== system umich_2d_walking/DAQ/OSU_to_CMU ==
  note: Order:
      |
      | backJointR
      | backGearR
      | frontJointR
      | frontGearR
      |
      | backJointL
      | backGearL
      | frontJointL
      | frontGearL
      |
      | latR
      | latL
      |
      | boomRoll
      | boomYaw
      | boomPitch
  q_osu : Inport
  q_initial : Inport  Port=2
  Constant : Constant  Value=3*pi/2
  Constant1 : Constant  Value=3*pi/2
  Constant2 : Constant  Value=3*pi/2
  Demux2 : Demux  Outputs=15
  Demux3 : Demux
  Mux1 : Mux  Inputs=8
  Mux23 : Mux  Inputs=6
  Sum : Sum  Inputs=+-|
  Sum1 : Sum  Inputs=-+|
  Sum2 : Sum  Inputs=+-|
  Sum3 : Sum  Inputs=++-
  Sum4 : Sum  Inputs=++-
  Terminator : Terminator
  Terminator1 : Terminator
  Terminator2 : Terminator
  reverse : Gain  Gain=-1
  signal : Gain  Gain=180/pi
  q : Outport
  wires:
  signal/1 -> Terminator2/1
  Mux23/1 -> signal/1, q/1
  [qLatL] -> Mux23/3
  [qLatR] -> Mux23/2
  [qLatR_inc_osu] -> Sum4/1
  [qLatL_inc_osu] -> Sum3/1
  Sum4/1 -> [qLatR]  "qLatR"
  Sum3/1 -> [qLatL]  "qLatL"
  Sum2/1 -> Mux23/1
  Mux1/1 -> Sum2/2
  Constant2/1 -> Sum2/1
  Demux2/6 -> Mux1/6  "qBackGearL_osu"
  Demux2/14 -> Mux23/5  "qBoomYaw"
  Demux2/8 -> Mux1/8  "qFrontGearL_osu"
  Demux3/3 -> Sum1/2  "qLatR_osu_abs_Initial"
  Demux2/3 -> Mux1/3  "qFrontR_osu"
  Demux2/5 -> Mux1/5  "qBackL_osu"
  Demux2/10 -> [qLatL_inc_osu]  "qLatL_inc_osu"
  Demux2/12 -> [qLatR_inc_osu]  "qLatR_inc_osu"
  Sum1/1 -> Sum4/2  "qLatR_abs_Initial"
  Sum/1 -> Sum3/2  "qLatL_abs_Initial"
  Demux2/1 -> Mux1/1  "qBackR_osu"
  q_osu/1 -> Demux2/1
  q_initial/1 -> Demux3/1
  Constant/1 -> Sum/1
  Demux2/7 -> Mux1/7  "qFrontL_osu"
  Demux2/11 -> Terminator1/1  "qLatR_abs_osu"
  Demux3/1 -> Sum/2  "qLatL_osu_abs_Initial"
  Demux2/2 -> Mux1/2  "qBackGearR_osu"
  Demux2/9 -> Terminator/1  "qLatL_abs_osu"
  Demux3/4 -> Sum4/3  "qLatR_inc_Initial"
  Demux2/13 -> Mux23/4  "qBoomRoll"
  Demux2/4 -> Mux1/4  "qFrontGearR_osu"
  Constant1/1 -> Sum1/1
  Demux3/2 -> Sum3/3  "qLatL_inc_Initial"
  Demux2/15 -> reverse/1  "qBoomPitch"
  reverse/1 -> Mux23/6

== system umich_2d_walking/DAQ/calibrate_and_convert_to_rad ==
  encoder_ticks : Inport
  Constant : Constant  Value=HIP_INC_ENCODER_RAD_PER_TICK
  Constant1 : Constant  Value=HIP_INC_ENCODER_RAD_PER_TICK
  Constant2 : Constant  Value=BOOM_YAW_ENCODER_RAD_PER_TICK
  Mux1 : Mux  Inputs=2
  Mux2 : Mux  Inputs=3
  Product : Product  RndMeth=Zero
  Selector2 : Selector  InputPortWidth=15  IndexOptions=Index vector (dialog)  Indices=[1 2 3 4 5 6 7 8 9 13 10 14 11 15 12]  OutputSizes=1
  calibrate_abs_encoder : Subsystem
  calibration_pt_radians : Subsystem
  calibration_pt_ticks : Subsystem
  select_abs : Selector  InputPortWidth=15  IndexOptions=Index vector (dialog)  Indices=[1 2 3 4 5 6 7 8 9 11 13 15]  OutputSizes=1
  select_inc : Selector  InputPortWidth=15  IndexOptions=Index vector (dialog)  Indices=[10 12 14]  OutputSizes=1
  ticks_to_radians_constants : Subsystem
  q_osu : Outport
  wires:
  Constant2/1 -> Mux2/3
  Constant1/1 -> Mux2/2
  Constant/1 -> Mux2/1
  Product/1 -> Mux1/2
  Mux2/1 -> Product/2
  select_inc/1 -> Product/1
  Selector2/1 -> q_osu/1
  Mux1/1 -> Selector2/1
  select_abs/1 -> calibrate_abs_encoder/1(encoder_ticks)
  calibrate_abs_encoder/1(angle [rad]) -> Mux1/1
  ticks_to_radians_constants/1(ticks_to_rad_constants) -> calibrate_abs_encoder/4(ticks_to_rad_const)
  calibration_pt_radians/1(calibration_pt [rad]) -> calibrate_abs_encoder/3(cal_pt_rad)
  calibration_pt_ticks/1(calibration_pt [ticks]) -> calibrate_abs_encoder/2(cal_pt_ticks)
  encoder_ticks/1 -> select_abs/1, select_inc/1

== system umich_2d_walking/DAQ/hold_initial_lateral_angles ==
  note: Time compare constant must be greater than
      | "Task start offsets" parameter in
      | EtherCAT Update Network Device block
  q_osu : Inport
  Clock : Clock
  Compare to const : simulink/Logic and Bit Operations/Compare To Constant  relop=<=  const=3  OutDataTypeStr=boolean
  Initial Lateral Hip Angles [rad] : Subsystem  TreatAsAtomicUnit=on
  Selector : Selector  InputPortWidth=15  IndexOptions=Index vector (dialog)  Indices=[9 10 11 12]  OutputSizes=1
  qLat_initial [absL incL absR incR] : Outport
  wires:
  Compare to const/1 -> Initial Lateral Hip Angles [rad]/Enable
  Initial Lateral Hip Angles [rad]/1(Out) -> qLat_initial [absL incL absR incR]/1
  Clock/1 -> Compare to const/1
  q_osu/1 -> Selector/1
  Selector/1 -> Initial Lateral Hip Angles [rad]/1(In)

== system umich_2d_walking/DAQ/low_pass_derivative ==
  q : Inport
  Gain1 : Gain  Gain=1/sample_time
  difference : simulink/Discrete/Difference  ICPrevInput=0.0  InputProcessing=Inherited  OutMin=[]  OutMax=[]  OutDataType=fixdt(1, 16)  OutScaling=2^-10  DoSatur=off
  single_pole_filter : DiscreteTransferFcn  Numerator=[(1-exp(-2*pi*fcut_velocity*sample_time)) 0]  Denominator=[1 -exp(-2*pi*fcut_velocity*sample_time)]  SampleTime=sample_time
  dq : Outport
  wires:
  difference/1 -> single_pole_filter/1
  q/1 -> Gain1/1
  Gain1/1 -> difference/1
  single_pole_filter/1 -> dq/1
